simulink model "vehicle_hostmodel_2022b_Vignesh"  (R2022b)
settings: Solver=VariableStepAuto  StartTime=0  StopTime=1000  RelTol=1e-3
model workspace (MAT data in the model file):
  finalint = 0
  firstWarning = 1
  originalScenarioChecksum = '114339432DE22364D47BB28FC96DC10C'
undefined symbols (not defined in the file): Acceleration, ActorID, AngularVelocity, cameraParams, curvature, DefaultGear, DEND_B, DEND_S, DEND_T, direction, DiscIntNeverNeededParam, driving, gradbp, L, LF, LR, m, matlabshared, MAX_BRAKE, MAX_STEER, MAX_TORQUE, MCAR, MIN_BRAKE, MIN_STEER, MIN_TORQUE, n, NUMD_B, NUMD_S, NUMD_T, Pitch, Pose, Position, psi_o, R, Roll, RRdamp, SceneInfo, sigbuilder_block, STEER_RATIO, stopSign_ID, Tdead, thetaRefs, TL_ID, trackingParams, TrackWidth, Ts, ts, Vdead, Velocity, WB, X_o, xRef2s, Y_o, Yaw, yRef2, yRef2s
libraries: drivingscenarioandsensors x11, simulink x10, roadrunnerscenario x9, slrealtimeutilitieslib x7, slrealtimeiplib x7, simulink_extras x5, drivingvehiclecontroller x3, trackingutilitieslib x3, robotalgslib x2, slpidlib x2, drivinglib x2, eeGeneralControl x1
(part 1 of 5)
settings Model: Creator=akshran  LastModifiedBy=giridhar.9a
settings DataIOCC: SignalLogging=off
settings DebuggingCC: UnconnectedInputMsg=warning  UnconnectedOutputMsg=warning  UnconnectedLineMsg=warning  UnderSpecifiedDimensionMsg=warning
settings ModelReferenceCC: EnableRefExpFcnMdlSchedulingChecks=on
settings RTWCC: DLArmComputeVersion=19.05

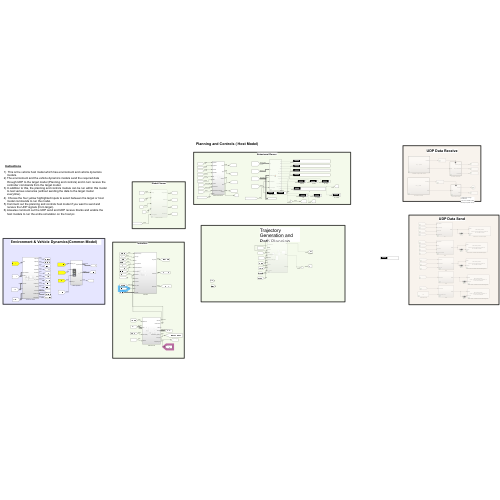
[thumbnail: Simulink's stored preview of the top-level diagram]
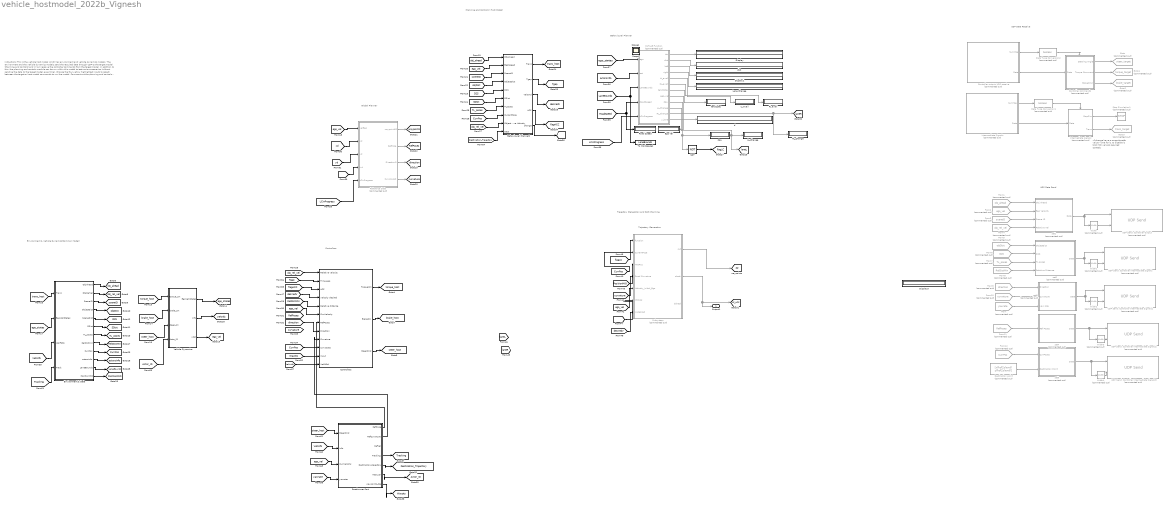
== system vehicle_hostmodel_2022b_Vignesh ==
  note: Trajectory Generation and Path Planning
  note: Global Planner
  note: xf change have a range
      | ttc safe value
      | - time for lc, to disable lc blok
      |
      | MIO vel pos required correctly
  note: Trajectory Generation
  note: Behavioural Planner
  note: Instructions
      |
      | This is the vehicle host model which has environment and vehicle dynamics models.
      | The environment and the vehicle dynamics models send the required data through UDP to the target model (Planning and controls) and in turn receive the controller commands from the target model.
      | In addition to this, the planning and controls module can be run within this model to test various scenarios (without sending the data to the target model everytime).
      | Choose the four yellow highlighted inputs to select between the target or host model commands to run the model.
      | Comment out the planning and controls host model if you want to send and receive the UDP signals (from target).
      | Likewise comment out the UDP send and UDP receive blocks and enable the host models to run the entire simulation on the host pc.
  note: Environment & Vehicle Dynamics(Common Model)
  note: UDP Data Receive
  note: UDP Data Send
  note: Planning and Controls ( Host Model)
  note: Controllers
  Behavioural Planner2 : Subsystem
  Controller commands : Subsystem  Commented=on
  Controller output- UDP receive : Subsystem  Commented=on
  Controllers : Subsystem
  Data Type Conversion1 : DataTypeConversion  Commented=on  OutDataTypeStr=boolean  SaturateOnIntegerOverflow=off  RndMeth=Floor
  Data Type Conversion2 : DataTypeConversion  Commented=on  OutDataTypeStr=boolean  SaturateOnIntegerOverflow=off  RndMeth=Floor
  Destination point : Constant  Commented=on  Value=[xRef2s(end) yRef2s(end)]
  Display : Display
  Display1 : Display
  Display3 : Display
  Ego Vel : Display
  Environment & Data : Subsystem
  From : From  Commented=on  GotoTag=yawrate  TagVisibility=global
  From1 : From  Commented=on  GotoTag=obj_ahead  TagVisibility=global
  From10 : From  Commented=on  GotoTag=curvature  TagVisibility=global
  From11 : From  Commented=on  GotoTag=RefPoses  TagVisibility=global
  From12 : From  Commented=on  GotoTag=CurrPos  TagVisibility=global
  From2 : From  Commented=on  GotoTag=ego_vel  TagVisibility=global
  From3 : From  Commented=on  GotoTag=sceneID  TagVisibility=global
  From4 : From  Commented=on  GotoTag=obj_rel_vel  TagVisibility=global
  From5 : From  Commented=on  GotoTag=objDist  TagVisibility=global
  From6 : From  Commented=on  GotoTag=D2S  TagVisibility=global
  From7 : From  Commented=on  GotoTag=TL_poses  TagVisibility=global
  From8 : From  Commented=on  GotoTag=RelDistMin  TagVisibility=global
  From9 : From  Commented=on  GotoTag=direction  TagVisibility=global
  Goto : Goto  Commented=on  GotoTag=steer_target  TagVisibility=global
  Goto1 : Goto  Commented=on  GotoTag=torque_target  TagVisibility=global
  Goto2 : Goto  Commented=on  GotoTag=brake_target  TagVisibility=global
  Goto3 : Goto  Commented=on  GotoTag=trans_target  TagVisibility=global
  Intermediate Signals : Subsystem  Commented=on
  Intermediate signals : Subsystem  Commented=on
  LL avail : Display
  LL_Change : Display
  "Lane Change " : Display
  MATLAB Function : MATLAB Function  Commented=on  TreatAsAtomicUnit=on
  NOT : Logic  Operator=NOT  IconShape=distinctive  AllPortsSameDT=off  OutDataTypeStr=boolean
  RL avail : Display
  RL_Change : Display
  Reference Data : Subsystem  Commented=on  VariantControl=Stanley
  Road Speed : Display
  Roadrunner Port : Subsystem
  Stop Simulation1 : Stop  Commented=on
  Subsystem : Subsystem  Commented=on
  To Workspace1 : ToWorkspace  VariableName=LaneBounds  SaveFormat=Timeseries  SampleTime=-1
  UDP Send: Controller Intermediate Signals : slrealtimeiplib/UDP Send  Commented=on  useHostTargetConn=on  toAddress=192.168.7.2  toPort=8002  sampleTime=0.1  enableMessage=off  ipAddress=192.168.7.2  localPort=-1
  UDP Send: Controller Intermediate Signals1 : slrealtimeiplib/UDP Send  Commented=on  useHostTargetConn=on  toAddress=192.168.7.2  toPort=8003  sampleTime=0.1  enableMessage=off  ipAddress=192.168.7.2  localPort=-1
  UDP Send: Controller Intermediate Signals2 : slrealtimeiplib/UDP Send  Commented=on  useHostTargetConn=on  toAddress=192.168.7.2  toPort=8004  sampleTime=0.1  enableMessage=off  ipAddress=192.168.7.2  localPort=-1
  UDP Send: Controller Intermediate Signals3 : slrealtimeiplib/UDP Send  Commented=on  useHostTargetConn=on  toAddress=192.168.7.2  toPort=8005  sampleTime=0.1  enableMessage=off  ipAddress=192.168.7.2  localPort=-1
  UDP Send: Controller Output : slrealtimeiplib/UDP Send  Commented=on  useHostTargetConn=on  toAddress=192.168.7.2  toPort=8001  sampleTime=0.1  enableMessage=off  ipAddress=192.168.7.2  localPort=-1
  Vehicle Dynamics : Subsystem
  Width{,1..4} (5 alike) : Width  Commented=on
  d : Display
  dist : Display
  set1 : Subsystem  Commented=on
  set2 : Subsystem  Commented=on
  set3 : Subsystem  Commented=on
  set4 : Subsystem  Commented=on
  set5 : Subsystem  Commented=on
  stay : Display
  tend2stay : Display
  Output1 : Outport
  Scope : Scope
  Scope1 : Scope
  tag scope: Actor_ID=global, CurrPos=global, D2S=global, Destination_Trajectory=global, LC_ACC=global, LaneBounds=global, PP=global, PositionMIO=global, RefPoses=global, RelDistMin=global, SDist=global, TL_poses=global, Tgap=global, Tracking=global, VehInfo=global, Waypts=global, actorsInfo=global, brake_host=global, curvature=global, desiredV=global, direction=global, ego_states=global, ego_vel=global, flagACC=global, flagLC=global, laneL=global, laneR=global, objDist=global, obj_ahead=global, obj_rel_vel=global, sceneID=global, steer_host=global, torque_host=global, trans_host=global, waypoints=global
  wires:
  Width/1 -> UDP Send: Controller Output/2
  Width1/1 -> UDP Send: Controller Intermediate Signals/2
  set1/1(Data) -> Width/1, UDP Send: Controller Output/1
  set2/1(Data) -> UDP Send: Controller Intermediate Signals/1, Width1/1
  set3/1(Data) -> UDP Send: Controller Intermediate Signals1/1, Width2/1
  Width2/1 -> UDP Send: Controller Intermediate Signals1/2
  Width3/1 -> UDP Send: Controller Intermediate Signals2/2
  set4/1(Data) -> Width3/1, UDP Send: Controller Intermediate Signals2/1
  set5/1(Data) -> Width4/1, UDP Send: Controller Intermediate Signals3/1
  Width4/1 -> UDP Send: Controller Intermediate Signals3/2
  From/1 -> set3/3(yaw rate)
  Controller output- UDP receive/2(Data) -> Controller commands/1(Data)
  Controller output- UDP receive/1(NumMsg) -> Data Type Conversion2/1
  Data Type Conversion2/1 -> Controller commands/Enable
  Data Type Conversion1/1 -> Intermediate signals/Enable
  Intermediate Signals/1(NumMsg) -> Data Type Conversion1/1
  Intermediate Signals/2(Data) -> Intermediate signals/1(Data)
  Intermediate signals/1(StopSim) -> Stop Simulation1/1
  Destination point/1 -> set5/2(Destination Point)
  Controller commands/1(Steering Angle) -> Goto/1
  Controller commands/2(Torque Command) -> Goto1/1
  Controller commands/3(BrakeCmd) -> Goto2/1
  Intermediate signals/2(Trans) -> Goto3/1
  Controllers/1(TorgueCm) -> [torque_host]
  Environment & Data/1(ObjAhead) -> [obj_ahead]
  Environment & Data/2(ObjRelVel) -> [obj_rel_vel]
  Environment & Data/3(SceneID) -> [sceneID]
  Environment & Data/4(ObjectDist) -> [objDist]
  Environment & Data/6(SDist) -> [SDist]
  Environment & Data/5(SceneDist) -> [D2S]
  Environment & Data/7(TL_poses) -> [TL_poses]
  Vehicle Dynamics/1(EgoVehStates) -> [ego_states]
  Vehicle Dynamics/3(xdot) -> [ego_vel]
  Environment & Data/8(RelDistmin) -> [RelDistMin]
  Vehicle Dynamics/2(Info) -> [VehInfo]
  From1/1 -> set1/1(Obj Ahead)
  From2/1 -> set1/2(Ego Velocity)
  From3/1 -> set1/3(Scene ID)
  From4/1 -> set1/4(Relative Vel)
  From5/1 -> set2/1(ObjectDist)
  From6/1 -> set2/2(D2S)
  From7/1 -> set2/3(TL poses)
  From8/1 -> set2/4(Relative Distance)
  From9/1 -> set3/1(Direction)
  From10/1 -> set3/2(Curvature)
  From11/1 -> set4/1(Ref Poses)
  From12/1 -> set5/1(CurrPoses)
  [torque_host] -> Vehicle Dynamics/1(torque_cm)
  [brake_host] -> Vehicle Dynamics/2(brake_cm)
  [steer_host] -> Vehicle Dynamics/3(steer_cm)
  [trans_host] -> Environment & Data/1(Trans)
  [ego_states] -> Environment & Data/2(EgoVehStates)
  [obj_rel_vel] -> Controllers/1(Relative velocity)
  [RelDistMin] -> Controllers/5(Relative distance)
  [ego_vel] -> Controllers/6(CurrVelocity)
  [direction] -> Controllers/8(Direction)
  [CurrPos] -> Controllers/10(curr poses)
  [VehInfo] -> Environment & Data/3(VehFdbk)
  Environment & Data/9(CurrPos) -> [CurrPos]
  Environment & Data/10(actorsinfo) -> [actorsInfo]
  [ego_states] -> MATLAB Function/1(ego)
  [actorsInfo] -> MATLAB Function/2(act)
  MATLAB Function/1(ttc) -> Display/1
  Environment & Data/11(LaneBounds) -> [LaneBounds]
  [LaneBounds] -> MATLAB Function/3(LaneBounds), To Workspace1/1
  MATLAB Function/3(left) -> Display1/1
  MATLAB Function/4(right) -> "Lane Change "/1
  MATLAB Function/2(dist) -> dist/1
  [RoadSpeed] -> Road Speed/1, MATLAB Function/4(RoadSpeed)
  MATLAB Function/8(ego_vel) -> Ego Vel/1
  MATLAB Function/6(RL_avail) -> RL avail/1
  MATLAB Function/5(LL_avail) -> LL avail/1
  MATLAB Function/7(tend2stay) -> tend2stay/1
  MATLAB Function/9(stay) -> NOT/1, stay/1
  MATLAB Function/10(LL_Change) -> LL_Change/1, [laneL]
  MATLAB Function/11(RL_Change) -> RL_Change/1, [laneR]
  MATLAB Function/12(y_lane) -> d/1
  Environment & Data/12(PositionMIO) -> [PositionMIO]
  NOT/1 -> [flagLC]
  [desiredV] -> Controllers/4(velocity desired)
  [ego_vel] -> Reference Data/1(velEgo)
  Reference Data/1(waypointPP) -> [waypoints]
  Reference Data/2(RefPose) -> [RefPoses]
  Reference Data/3(DirectionO) -> [direction]
  [xd] -> Reference Data/2(xd)
  [yd] -> Reference Data/3(yd)
  [Waypts] -> Controllers/11(Input)
  Reference Data/4(CurvatureO) -> [curvature]
  [LCinProgress] -> Reference Data/5(LCinProgress)
  [Tgap] -> Controllers/2(Time gap)
  [flagACC] -> Controllers/3(ACC)
  [LCinProgress] -> MATLAB Function/5(LCinProgress)
  [VehInfo] -> Controllers/12(VehFdbk)
  [sceneID] -> Behavioural Planner2/3(SceneID)
  [objDist] -> Behavioural Planner2/4(ObjectDist)
  [D2S] -> Behavioural Planner2/5(D2S)
  [CurrPos] -> Behavioural Planner2/8(CurrentPose)
  [obj_ahead] -> Behavioural Planner2/1(ObjAhead)
  [ego_vel] -> Behavioural Planner2/2(EgoSpeed)
  [SDist] -> Behavioural Planner2/6(SDist)
  [TL_poses] -> Behavioural Planner2/7(TLposes)
  [obj_rel_vel] -> Behavioural Planner2/9(Object Relative Velocity)
  Behavioural Planner2/1(Trans) -> [trans_host]
  Behavioural Planner2/2(Tgap) -> [Tgap]
  Behavioural Planner2/3(VelCmd) -> [desiredV]
  Behavioural Planner2/4(ACC) -> [flagACC]
  Behavioural Planner2/5(change) -> [change]
  [change] -> Reference Data/4(In4)
  Controllers/2(BrakeCm) -> [brake_host]
  Controllers/3(SteerCmd) -> [steer_host]
  [flagLC] -> Subsystem/1(function)
  [CurrPos] -> Subsystem/2(CurrentPose)
  [PositionMIO] -> Subsystem/3(MIOPos)
  [curvature] -> Subsystem/4(Road Curvature)
  [ego_vel] -> Subsystem/5(Velocity_Initial_Ego)
  [obj_rel_vel] -> Subsystem/6(MIOVel)
  [desiredV] -> Subsystem/7(V_desired)
  Subsystem/1(out) -> [PP]
  Subsystem/2(check) -> Output1/1, [LC_ACC]
  [VehInfo] -> Roadrunner Port/2(Info)
  [steer_host] -> Roadrunner Port/1(SteerCmd)
  Roadrunner Port/4(Tracking) -> [Tracking]
  [ego_vel] -> Roadrunner Port/3(CurrVelocity)
  [yawrate] -> Roadrunner Port/4(yawrate)
  Roadrunner Port/2(RefCurvature) -> Controllers/9(Curvature)
  Roadrunner Port/1(RefPose) -> Controllers/7(RefPoses)
  [Tracking] -> Environment & Data/4(Track)
  Roadrunner Port/5(Destination_trajectory) -> [Destination_Trajectory]
  [Destination_Trajectory] -> Behavioural Planner2/10(Dest)
  Roadrunner Port/6(Actor_ID) -> [Actor_ID]
  [Actor_ID] -> Vehicle Dynamics/4(Actor_ID)
  Roadrunner Port/7(waypoints_traj) -> [Waypts]

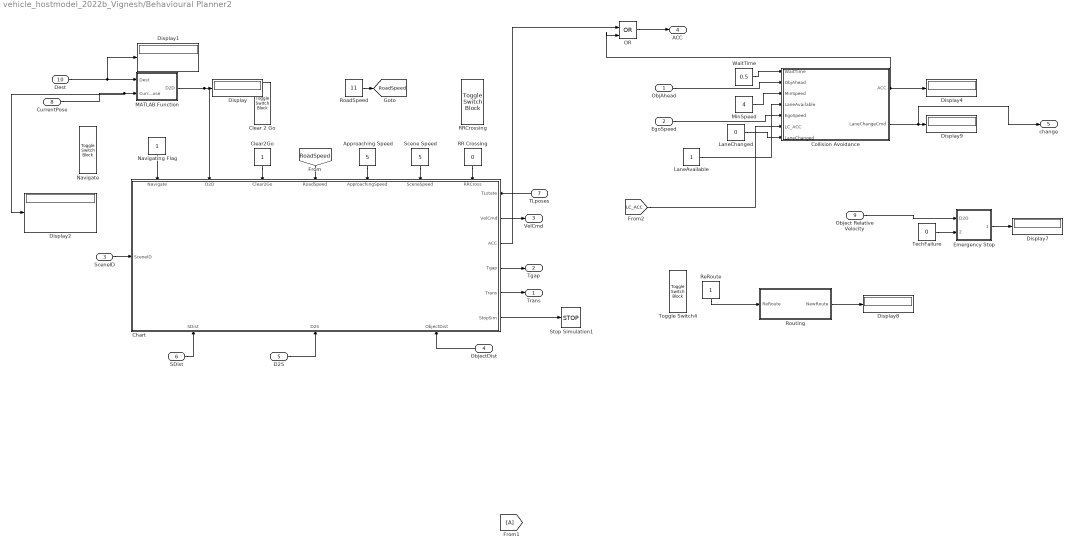
== system vehicle_hostmodel_2022b_Vignesh/Behavioural Planner2 ==
  ObjAhead : Inport
  EgoSpeed : Inport  Port=2
  SceneID : Inport  Port=3
  ObjectDist : Inport  Port=4
  D2S : Inport  Port=5
  SDist : Inport  Port=6
  TLposes : Inport  Port=7
  CurrentPose : Inport  Port=8
  Object Relative Velocity : Inport  Port=9
  Dest : Inport  Port=10
  Approaching Speed : Constant  Value=5
  Chart : Stateflow chart  TreatAsAtomicUnit=on
      settings: PortSchema="{\"entries\":[{\"content\":{\"sides\":[{\"content\":{\"connectorIds\":[\"In12\"]},\"type\":\"ConnectorPlacement.EquallySpacedRectSide\",\"uuid\":\"81aca70f-0947-49fb-b60a-be241e44193b\"},{\"content\":{\"connectorIds\":[\"In1\",\"Out1\",\"Out2\",\"Out3\",\"Out4\",\"Out5\"],\"side\":\"RIGHT\"},\"type\":\"ConnectorPlacement.EquallySpacedRectSide\",\"uuid\":\"e7b9645e-3711-4964-ac9b-0199dd335e99\"},{\"content\":{\"connectorIds\":[\"In8\",\"In9\",\"In10\",\"In11\",\"In2\",\"In4\",\"In6\"],\"side\":\"TOP\"},\"type\":\"ConnectorPlacement.EquallySpacedRectSide\",\"uuid\":\"6876f024-944b-4540-9404-d68f37763657\"},{\"content\":{\"connectorIds\":[\"In5\",\"In7\",\"In3\"],\"side\":\"BOTTOM\"},\"type\":\"ConnectorPlacement.EquallySpacedRectSide\",\"uuid\":\"44acab73-cdde-4edf-95df-27422644ccab\"}]},\"type\":\"ConnectorPlacement.EquallySpacedConnector\",\"uuid\":\"d2c31c01-e447-43db-8d2b-8b98a0ca291a\"}],\"packageUris\":[\"http://schema.mathworks.com/mf0/Connector/R2020b\"],\"version\":\"1.0\"}"
  Clear 2 Go : ToggleSwitchBlock
      settings: Values={{'Off', 'On'}, [0 1]}
  Clear2Go : Constant
  Collision Avoidance : Stateflow chart  TreatAsAtomicUnit=on
  Display{,1..2,4,7..9} (7 alike) : Display
  Emergency Stop : Stateflow chart  TreatAsAtomicUnit=on
  From1 : From
  LaneAvailable : Constant
  LaneChanged : Constant  Value=0
  MATLAB Function : MATLAB Function  TreatAsAtomicUnit=on
  MinSpeed : Constant  Value=4
  Navigate : ToggleSwitchBlock
      settings: Values={{'Off', 'On'}, [0 1]}
  Navigating Flag : Constant
  OR : Logic  Operator=OR  IconShape=distinctive  AllPortsSameDT=off  OutDataTypeStr=fixdt(1,16)
  RR Crossing : Constant  Value=0
  RRCrossing : ToggleSwitchBlock
      settings: Values={{'Off', 'On'}, [0 1]}
  ReRoute : Constant
  RoadSpeed : Constant  Value=11
  Routing : Stateflow chart  TreatAsAtomicUnit=on
  Scene Speed : Constant  Value=5
  Stop Simulation1 : Stop
  TechFailure : Constant  Value=0
  Toggle Switch4 : ToggleSwitchBlock
      settings: Values={{'Off', 'On'}, [0 1]}
  WaitTime : Constant  Value=0.5
  Trans : Outport
  Tgap : Outport  Port=2
  VelCmd : Outport  Port=3
  ACC : Outport  Port=4
  change : Outport  Port=5
  tag scope: RoadSpeed=global
  wires:
  Clear2Go/1 -> Chart/10(Clear2Go)
  Routing/1(NewRoute) -> Display8/1
  ObjectDist/1 -> Chart/3(ObjectDist)
  WaitTime/1 -> Collision Avoidance/1(WaitTime)
  Navigating Flag/1 -> Chart/8(Navigate)
  Approaching Speed/1 -> Chart/2(ApproachingSpeed)
  Scene Speed/1 -> Chart/4(SceneSpeed)
  EgoSpeed/1 -> Collision Avoidance/5(EgoSpeed)
  ReRoute/1 -> Routing/1(ReRoute)
  Collision Avoidance/2(LaneChangeCmd) -> change/1, Display9/1
  LaneAvailable/1 -> Collision Avoidance/4(LaneAvailable)
  CurrentPose/1 -> Display2/1, MATLAB Function/2(CurrentPose)
  RR Crossing/1 -> Chart/6(RRCross)
  MinSpeed/1 -> Collision Avoidance/3(MinSpeed)
  LaneChanged/1 -> Collision Avoidance/7(LaneChanged)
  [RoadSpeed] -> Chart/11(RoadSpeed)
  ObjAhead/1 -> Collision Avoidance/2(ObjAhead)
  Dest/1 -> Display1/1, MATLAB Function/1(Dest)
  SceneID/1 -> Chart/12(SceneID)
  MATLAB Function/1(D2D) -> Display/1, Chart/9(D2D)
  Chart/5(StopSim) -> Stop Simulation1/1
  Chart/4(Trans) -> Trans/1
  TLposes/1 -> Chart/1(TLstate)
  Chart/1(VelCmd) -> VelCmd/1
  SDist/1 -> Chart/5(SDist)
  D2S/1 -> Chart/7(D2S)
  Chart/3(Tgap) -> Tgap/1
  TechFailure/1 -> Emergency Stop/2(TechFailure)
  Emergency Stop/1(EStop) -> Display7/1
  Object Relative Velocity/1 -> Emergency Stop/1(D2O)
  Collision Avoidance/1(ACC) -> OR/2, Display4/1
  OR/1 -> ACC/1
  Chart/2(ACC) -> OR/1
  RoadSpeed/1 -> [RoadSpeed]
  [LC_ACC] -> Collision Avoidance/6(LC_ACC)

== system vehicle_hostmodel_2022b_Vignesh/Controller commands ==
  Data : Inport
  Enable : EnablePort
  "Byte Unpacking " : slrealtimeutilitieslib/Byte Unpacking  MaskUnpackedDataTypes={'double', 'double', 'double'}  MaskUnpackedDataSizes={[1], [1], [1]}  MaskAlignment=1
  Steering Angle : Outport
  Torque Command : Outport  Port=2
  BrakeCmd : Outport  Port=3
  wires:
  Data/1 -> "Byte Unpacking "/1
  "Byte Unpacking "/1 -> Steering Angle/1  "Steering angle"
  "Byte Unpacking "/2 -> Torque Command/1  "Longitudinal velocity"
  "Byte Unpacking "/3 -> BrakeCmd/1  "BrakeCmd"

== system vehicle_hostmodel_2022b_Vignesh/Controller output- UDP receive ==
  Compare To Constant : simulink/Logic and Bit Operations/Compare To Constant  relop===  const=24  OutDataTypeStr=boolean
  Constant : Constant
  Subtract : Sum  Inputs=+-
  UDP Receive2 : slrealtimeiplib/UDP Receive  useHostTargetConn=on  ipAddress=192.168.7.2  localPort=8016  rcvWidth=24  rcvFmAny=off  fmAddress=192.168.7.2  sampleTime=-1  enableMessage=off  maxPackets=1
  While Iterator : WhileIterator  WhileBlockType=do-while  ResetStates=reset  ShowIterationPort=on
  NumMsg : Outport
  Data : Outport  Port=2
  wires:
  Compare To Constant/1 -> While Iterator/1
  UDP Receive2/1 -> Data/1
  Constant/1 -> Subtract/2
  Subtract/1 -> NumMsg/1
  UDP Receive2/2 -> Compare To Constant/1
  While Iterator/1 -> Subtract/1

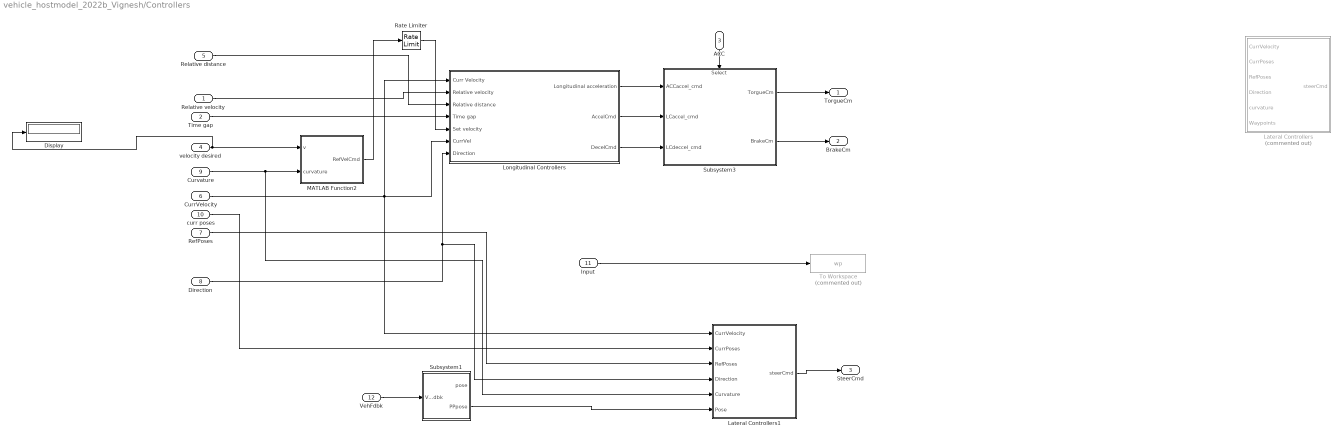
== system vehicle_hostmodel_2022b_Vignesh/Controllers ==
  Relative velocity : Inport
  Time gap : Inport  Port=2
  ACC : Inport  Port=3
  velocity desired : Inport  Port=4
  Relative distance : Inport  Port=5
  CurrVelocity : Inport  Port=6
  RefPoses : Inport  Port=7
  Direction : Inport  Port=8
  Curvature : Inport  Port=9
  curr poses : Inport  Port=10
  Input : Inport  Port=11
  VehFdbk : Inport  Port=12
  Display : Display
  Lateral Controllers : Subsystem  Commented=on
  Lateral Controllers1 : Subsystem
  Longitudinal Controllers : Subsystem
  MATLAB Function2 : MATLAB Function  TreatAsAtomicUnit=on
  Rate Limiter : RateLimiter  RisingSlewLimit=2  SampleTimeMode=inherited
  Subsystem1 : Subsystem
  Subsystem3 : Subsystem
      settings: PortSchema="{\"entries\":[{\"content\":{\"sides\":[{\"content\":{\"connectorIds\":[\"In1\",\"In2\",\"In3\"]},\"type\":\"ConnectorPlacement.EquallySpacedRectSide\",\"uuid\":\"a23b1a10-3bcb-40a0-900c-c9a3f160b173\"},{\"content\":{\"connectorIds\":[\"Out1\",\"Out2\"],\"side\":\"RIGHT\"},\"type\":\"ConnectorPlacement.EquallySpacedRectSide\",\"uuid\":\"88840b66-912f-4184-aeec-297642319416\"},{\"content\":{\"connectorIds\":[\"In4\"],\"side\":\"TOP\"},\"type\":\"ConnectorPlacement.EquallySpacedRectSide\",\"uuid\":\"37a03ca9-b065-473e-b290-3b07703c6005\"}]},\"type\":\"ConnectorPlacement.EquallySpacedConnector\",\"uuid\":\"5bfc7c71-8f7a-4cba-a168-7eeca22a2fcb\"}],\"packageUris\":[\"http://schema.mathworks.com/mf0/Connector/R2020b\"],\"version\":\"1.0\"}"
  To Workspace : ToWorkspace  Commented=on  VariableName=wp  SampleTime=-1
  TorgueCm : Outport
  BrakeCm : Outport  Port=2
  SteerCmd : Outport  Port=3
  wires:
  Longitudinal Controllers/1(Longitudinal acceleration) -> Subsystem3/1(ACCaccel_cmd)
  Curvature/1 -> MATLAB Function2/2(curvature), Lateral Controllers1/5(Curvature)
  Relative velocity/1 -> Longitudinal Controllers/2(Relative velocity)
  MATLAB Function2/1(RefVelCmd) -> Rate Limiter/1
  Direction/1 -> Longitudinal Controllers/7(Direction), Lateral Controllers1/4(Direction)
  RefPoses/1 -> Lateral Controllers1/3(RefPoses)
  velocity desired/1 -> Display/1, MATLAB Function2/1(v)
  Longitudinal Controllers/2(AccelCmd) -> Subsystem3/2(LCaccel_cmd)
  Longitudinal Controllers/3(DecelCmd) -> Subsystem3/3(LCdeccel_cmd)
  CurrVelocity/1 -> Longitudinal Controllers/1(Curr Velocity), Longitudinal Controllers/6(CurrVel), Lateral Controllers1/1(CurrVelocity)
  Time gap/1 -> Longitudinal Controllers/4(Time gap)
  Relative distance/1 -> Longitudinal Controllers/3(Relative distance)
  ACC/1 -> Subsystem3/4(Select)
  Subsystem3/1(TorgueCm) -> TorgueCm/1
  Subsystem3/2(BrakeCm) -> BrakeCm/1
  Input/1 -> To Workspace/1
  Subsystem1/2(PPpose) -> Lateral Controllers1/6(Pose)
  VehFdbk/1 -> Subsystem1/1(VehFdbk)
  Lateral Controllers1/1(steerCmd) -> SteerCmd/1
  Rate Limiter/1 -> Longitudinal Controllers/5(Set velocity)
  curr poses/1 -> Lateral Controllers1/2(CurrPoses)

== system vehicle_hostmodel_2022b_Vignesh/Environment & Data ==
  Trans : Inport
  EgoVehStates : Inport  Port=2
  VehFdbk : Inport  Port=3
  Track : Inport  Port=4
  Bus Selector4 : BusSelector  OutputSignals=Velocity,Acceleration,Position
  Sensors & Perception : Subsystem
  Subsystem1 : Subsystem
  Terminator1 : Terminator
  Terminator2 : Terminator
  Terminator3 : Terminator
  Visualisation & Data : Subsystem
  ObjAhead : Outport
  ObjRelVel : Outport  Port=2
  SceneID : Outport  Port=3
  ObjectDist : Outport  Port=4
  SceneDist : Outport  Port=5
  SDist : Outport  Port=6
  TL_poses : Outport  Port=7
  RelDistmin : Outport  Port=8
  CurrPos : Outport  Port=9
  actorsinfo : Outport  Port=10
  LaneBounds : Outport  Port=11
  PositionMIO : Outport  Port=12
  wires:
  Bus Selector4/3 -> Visualisation & Data/4(Ego Position)  "<Position>"
  Sensors & Perception/1(ObjAhead) -> ObjAhead/1
  Bus Selector4/1 -> Visualisation & Data/2(EgoVelocity)  "<Velocity>"
  Visualisation & Data/1(Actors_VehCoords) -> Sensors & Perception/1(Detections)
  Sensors & Perception/5(SceneRelVel) -> Terminator2/1
  Sensors & Perception/2(SceneAhead) -> Terminator1/1
  Sensors & Perception/6(ObjectDist) -> ObjectDist/1
  Bus Selector4/2 -> Visualisation & Data/3(Ego Acceleration)  "<Acceleration>"
  Sensors & Perception/9(ReVelmin) -> Terminator3/1
  EgoVehStates/1 -> Visualisation & Data/5(EgoInfo), Visualisation & Data/1(EgoVehStates), Sensors & Perception/2(EgoInfo), Bus Selector4/1
  Sensors & Perception/4(ObjRelVel) -> ObjRelVel/1
  Visualisation & Data/2(TL_poses) -> TL_poses/1
  Sensors & Perception/3(SceneID) -> SceneID/1
  Sensors & Perception/8(SDist) -> SDist/1
  Sensors & Perception/7(SceneDist) -> SceneDist/1
  Trans/1 -> Sensors & Perception/4(Trans)
  Sensors & Perception/10(RelDistmin) -> RelDistmin/1
  VehFdbk/1 -> Subsystem1/1(VehFdbk)
  Subsystem1/1(pose) -> CurrPos/1
  Visualisation & Data/3(actorsinfo) -> actorsinfo/1
  Visualisation & Data/4(LaneBounds) -> LaneBounds/1, Sensors & Perception/3(LaneBounds)
  Sensors & Perception/11(PositionMIO) -> PositionMIO/1
  Track/1 -> Sensors & Perception/5(Track)

== system vehicle_hostmodel_2022b_Vignesh/Intermediate Signals ==
  Compare To Constant : simulink/Logic and Bit Operations/Compare To Constant  relop===  const=16  OutDataTypeStr=boolean
  Constant : Constant
  Subtract : Sum  Inputs=+-
  UDP Receive2 : slrealtimeiplib/UDP Receive  useHostTargetConn=on  ipAddress=192.168.7.2  localPort=8017  rcvWidth=16  rcvFmAny=off  fmAddress=192.168.7.2  sampleTime=-1  enableMessage=off  maxPackets=1
  While Iterator : WhileIterator  WhileBlockType=do-while  ResetStates=reset  ShowIterationPort=on
  NumMsg : Outport
  Data : Outport  Port=2
  wires:
  While Iterator/1 -> Subtract/1
  UDP Receive2/2 -> Compare To Constant/1
  Subtract/1 -> NumMsg/1
  Constant/1 -> Subtract/2
  UDP Receive2/1 -> Data/1
  Compare To Constant/1 -> While Iterator/1

== system vehicle_hostmodel_2022b_Vignesh/Intermediate signals ==
  Data : Inport
  Enable : EnablePort
  "Byte Unpacking " : slrealtimeutilitieslib/Byte Unpacking  MaskUnpackedDataTypes={'double', 'double'}  MaskUnpackedDataSizes={[1], [1]}  MaskAlignment=1
  StopSim : Outport
  Trans : Outport  Port=2
  wires:
  "Byte Unpacking "/2 -> Trans/1  "Trans"
  "Byte Unpacking "/1 -> StopSim/1  "StopSim"
  Data/1 -> "Byte Unpacking "/1

== system vehicle_hostmodel_2022b_Vignesh/Reference Data ==
  velEgo : Inport
  xd : Inport  Port=2
  yd : Inport  Port=3
  In4 : Inport  Port=4
  LCinProgress : Inport  Port=5
  Discrete-Time Integrator : DiscreteIntegrator  SampleTime=-1  ICPrevOutput=DiscIntNeverNeededParam  ICPrevScaledInput=DiscIntNeverNeededParam
  Memory : Memory
  Memory1 : Memory
  Merge : Merge
  Merge1 : Merge
  Subsystem : Subsystem
  Subsystem1 : Subsystem
  Subsystem2 : Subsystem
  Subsystem3 : Subsystem
  Switch : Switch  Criteria=u2 ~= 0  SaturateOnIntegerOverflow=off  InputSameDT=off
  Switch Case : SwitchCase  CaseConditions={1,0}  ShowDefaultCase=off
  waypointPP : Outport
  RefPose : Outport  Port=2
  DirectionO : Outport  Port=3
  CurvatureO : Outport  Port=4
  wires:
  velEgo/1 -> Subsystem3/1(VelFdbk), Subsystem2/1(VelFdbk), Discrete-Time Integrator/1
  Subsystem2/4(WayPoints) -> Merge1/1
  Merge1/1 -> waypointPP/1
  Subsystem2/1(RefPose) -> Switch/3
  Subsystem2/2(DirectionO) -> DirectionO/1
  Merge/1 -> CurvatureO/1
  Subsystem2/3(CurvatureO) -> Merge/2
  Subsystem3/1(RefPose) -> Switch/1
  Switch Case/1 -> Subsystem3/Action
  Switch Case/2 -> Subsystem2/Action
  xd/1 -> Memory/1
  yd/1 -> Memory1/1
  Memory/1 -> Subsystem3/2(xd)
  Memory1/1 -> Subsystem3/4(yd)
  Subsystem2/5(finalint) -> Subsystem3/3(finalint)
  Subsystem/1(Out1) -> Switch/2, Switch Case/1, Subsystem1/2(enable)
  LCinProgress/1 -> Subsystem/Enable
  Discrete-Time Integrator/1 -> Subsystem1/1(Integrator)
  Subsystem1/1(Ref pose) -> RefPose/1

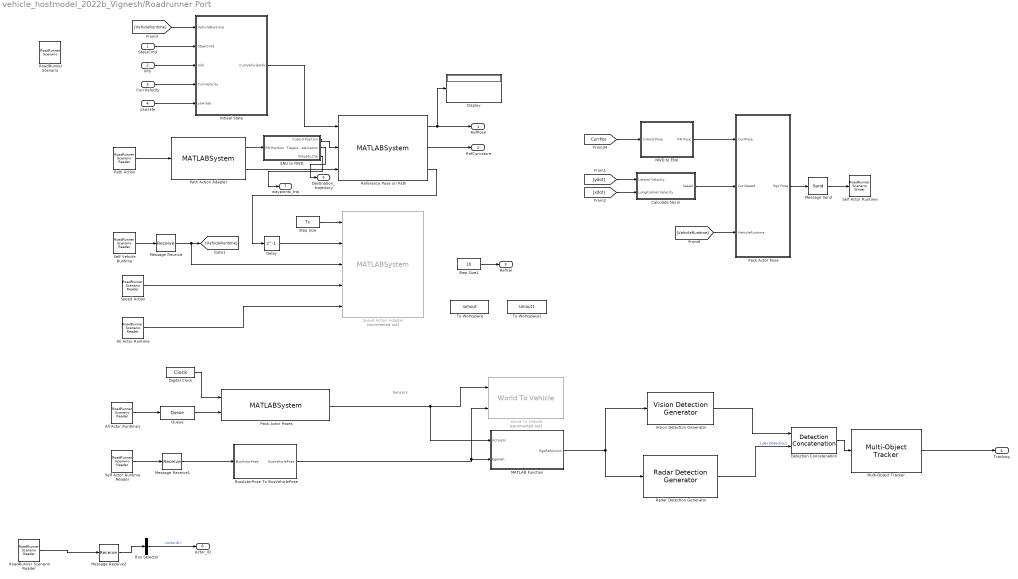
== system vehicle_hostmodel_2022b_Vignesh/Roadrunner Port ==
  note: Sensors
  SteerCmd : Inport
  Info : Inport  Port=2
  CurrVelocity : Inport  Port=3
  yawrate : Inport  Port=4
  All Actor Runtime : roadrunnerscenario/RoadRunner Scenario Reader  TopicCategory=Actor  ActorCategory=All Types  ActionType=Path Following  TopicType=Actor Pose  VehicleType=Vehicle Specifications  UserDefinedAction=Action1  Filter=None  SampleTime=Ts
  All Actor Runtime1 : roadrunnerscenario/RoadRunner Scenario Reader  TopicCategory=Actor  ActorCategory=All Types  ActionType=Path Following  TopicType=Actor Pose (Driving Scenario compatible)  VehicleType=Vehicle Specifications  UserDefinedAction=Action1  Filter=None  SampleTime=Ts
  Bus Selector : BusSelector  OutputSignals=ActorID
  BusActorPose To BusVehiclePose : Subsystem
  Calculate Norm : Subsystem
  Delay : Delay  DelayLength=1  InitialCondition=logical(0)
  Detection Concatenation : trackingutilitieslib/Detection Concatenation  NumInputs=2  BusNameSource=Auto  BusName=BusDetectionConcatenation  SimulateUsing=Code generation
  Digital Clock : DigitalClock  SampleTime=Ts
  Display : Display
  ENU to NWD : Subsystem
  Initiaal State : Subsystem
  MATLAB Function : MATLAB Function  TreatAsAtomicUnit=on
  Message Receive : Receive  InputPortMessageModes=m
  Message Receive1 : Receive  InputPortMessageModes=m  SampleTime=Ts
  Message Receive2 : Receive  InputPortMessageModes=m  SampleTime=Ts
  Message Send : Send  OutputPortMessageModes=m
  Multi-Object Tracker : drivinglib/Multi-Object Tracker  TrackerIndex=uint32( 0 )  FilterInitializationFcn=initcvekf  AssignmentThreshold=trackingParams.assigThresh  ConfirmationThreshold=[trackingParams.M,trackingParams.N]  DeletionThreshold=[trackingParams.numCoasts,trackingParams.numCoasts]  MaxNumTracks=trackingParams.numTracks  MaxNumSensors=trackingParams.numSensors  OOSMHandling=Terminate  StateParametersSimulink=struct  HasStateParametersInput=off  TimeInputSource=Auto  HasCostMatrixInput=off  HasDetectableTrackIDsInput=off  BusNameSource=Property  BusName=BusMultiObjectTracker1  TentativeTracksOutputPort=off  AllTracksOutputPort=off  SimulateUsing=Interpreted execution
  NWD to ENU : Subsystem
  Pack Actor Pose : Subsystem
  Pack Actor Poses : MATLABSystem  InputPortMessageModes=n,m  System=HelperPackDrivingScenarioPoses  EgoActorID=1  ActorProfiles=struct( 'ActorID', 1, 'ClassID', 1, 'Length', 4.7, 'Width', 1.8, 'Height', 1.4, 'OriginOffset', [ 0, 0, 0 ], 'FrontOverhang', 0, 'RearOverhang', 0, 'Wheelbase', 0, 'Color', [ 0, 0, 0 ] )  DefaultActorPoses="Simulink.Bus.createMATLABStruct( \"BusActors\" )"
      mask Type: HelperPackDrivingScenarioPoses
      mask Display:
      | disp(['HelperPack' char(10) 'DrivingScenarioPoses']);
      | port_label('input',1,'time');
      | port_label('input',2,'msgs');
      | port_label('output',1,'TargetPoses');
  Path Action : roadrunnerscenario/RoadRunner Scenario Reader  TopicCategory=Action  ActorCategory=All Types  ActionType=Path Following  TopicType=Actor Specifications  VehicleType=Vehicle Specifications  UserDefinedAction=Action1  Filter=Self  SampleTime=Ts
  Path Action Adapter : MATLABSystem  InputPortMessageModes=m  System=HelperPathActionAdapter
      mask Type: HelperPathActionAdapter
      mask Display:
      | disp(['HelperPathActionAdapter' char(10) '' char(10) '']);
      | port_label('input',1,'PathAction');
      | port_label('output',1,'Path');
      | port_label('output',2,'NumPoints');
  Queue : Queue  InputPortMessageModes=m  OutputPortMessageModes=m  OverwriteOldest=on  Capacity=maxNumActors
  Radar Detection Generator : drivingscenarioandsensors/Radar Detection Generator  SensorIndex=2  UpdateInterval=0.01  SensorLocation=[ 1.5, 0 ]  Height=0.2  Yaw=0  Pitch=0  Roll=0  BusNameSource=Auto  BusName=BusRadarDetectionGenerator  MaxNumDetectionsSource=Property  MaxNumDetections=50  DetectionCoordinates=Ego Cartesian  SimulateUsing=Interpreted execution  AzimuthResolution=4  ElevationResolution=10  RangeResolution=2.5  RangeRateResolution=0.5  AzimuthBiasFraction=0.1  ElevationBiasFraction=0.1  RangeBiasFraction=0.05  RangeRateBiasFraction=0.05  FieldOfView=[ 60, 5 ]  MaxRange=150  RangeRateLimits=[ -100, 100 ]  DetectionProbability=0.9  FalseAlarmRate=1e-6  ReferenceRange=100  ReferenceRCS=0  HasElevation=off  HasRangeRate=on  HasNoise=on  HasFalseAlarms=on  HasOcclusion=on  InitialSeedSource=Repeatable  InitialSeed=0  UsedSeed=matlabshared.tracking.internal.SimulinkUtilities.seedManager(gcb)  ActorProfilesSource=Parameters  ActorProfilesParameters=driving.internal.ActorProfilesRadarParameters  ActorProfilesExpression=struct( 'ClassID', 0, 'Length', 4.7, 'Width', 1.8, 'Height', 1.4, 'OriginOffset', [ -1.35, 0, 0 ], 'RCSPattern', [ 10, 10; 10, 10 ], 'RCSAzimuthAngles', [ -180, 180 ], 'RCSElevationAngles', [ -90, 90 ] )
  Reference Pose on Path : MATLABSystem  System=HelperReferencePoseOnPath
      mask Type: HelperReferencePoseOnPath
      mask Display:
      | disp(['HelperReferencePoseOnPath' char(10) '' char(10) '' char(10) '' char(10) '']);
      | port_label('input',1,'PrevVehicleInfo');
      | port_label('input',2,'Trajectory');
      | port_label('input',3,'NumTrajPoints');
      | port_label('output',1,'RefPointOnPath');
      | port_label('output',2,'RefCurvature');
      | port_label('output',3,'IsGoalReached');
  RoadRunner Scenario : roadrunnerscenario/RoadRunner Scenario  UserDefinedActions={}
  RoadRunner Scenario Reader : roadrunnerscenario/RoadRunner Scenario Reader  TopicCategory=Actor  ActorCategory=All Types  ActionType=Path Following  TopicType=Actor Specifications  VehicleType=Vehicle Specifications  UserDefinedAction=Action1  Filter=Self  SampleTime=0
  Self Actor Runtime : roadrunnerscenario/RoadRunner Scenario Writer  TopicCategory=Actor  ActorCategory=All Types  EventType=Action Complete  VehicleType=Vehicle Pose  TopicType=Actor Pose
  Self Actor Runtime Reader : roadrunnerscenario/RoadRunner Scenario Reader  TopicCategory=Actor  ActorCategory=All Types  ActionType=Path Following  TopicType=Actor Pose (Driving Scenario compatible)  VehicleType=Vehicle Specifications  UserDefinedAction=Action1  Filter=Self  SampleTime=Ts
  Self Vehicle Runtime : roadrunnerscenario/RoadRunner Scenario Reader  TopicCategory=Actor  ActorCategory=Vehicle  ActionType=Path Following  TopicType=Actor Specifications  VehicleType=Vehicle Pose  UserDefinedAction=Action1  Filter=Self  SampleTime=Ts
  Speed Action : roadrunnerscenario/RoadRunner Scenario Reader  TopicCategory=Action  ActorCategory=All Types  ActionType=Speed Change  TopicType=Actor Specifications  VehicleType=Vehicle Specifications  UserDefinedAction=Action1  Filter=Self  SampleTime=Ts
  Speed Action Adapter : MATLABSystem  Commented=on  InputPortMessageModes=n,n,n,m,m  System=HelperSpeedActionAdapter
      mask Type: HelperSpeedActionAdapter
      mask Display:
      | disp(['HelperSpeedActionAdapter' char(10) '' char(10) '']);
      | port_label('input',1,'timestep');
      | port_label('input',2,'stopVehicle');
      | port_label('input',3,'vehicleRuntime');
      | port_label('input',4,'msgSpeedAction');
      | port_label('input',5,'msgAllVehicleRuntime');
      | port_label('output',1,'currentSpeed');
  Step Size : Constant  Value=Ts
  Step Size1 : Constant  Value=10
  To Workspace : ToWorkspace  VariableName=simout  SaveFormat=Timeseries  SampleTime=-1
  To Workspace1 : ToWorkspace  VariableName=simout1  SaveFormat=Timeseries  SampleTime=-1
  Vision Detection Generator : drivingscenarioandsensors/Vision Detection Generator  SensorIndex=1  DetectorOutput=Objects only  UpdateInterval=Ts  LaneUpdateInterval=Ts  SensorLocation=[ 2.1, 0 ]  Height=1.1  Yaw=0  Pitch=cameraParams.pitchAngle  Roll=0  BusNameSource=Auto  BusName=BusVision  BusName2Source=Auto  BusName2=BusLaneDetections  MaxNumDetectionsSource=Property  MaxNumDetections=20  MaxNumLanesSource=Property  MaxNumLanes=30  DetectionCoordinates=Ego Cartesian  SimulateUsing=Interpreted execution  MaxRange=cameraParams.cameraRange  BoundingBoxAccuracy=5  ProcessNoiseIntensity=5  MaxSpeed=50  MaxAllowedOcclusion=0.5  MinObjectImageSize=[ 15, 15 ]  DetectionProbability=0.9  FalsePositivesPerImage=0.1  MinLaneImageSize=[ 20, 5 ]  LaneBoundaryAccuracy=3  HasNoise=on  InitialSeedSource=Repeatable  InitialSeed=0  UsedSeed=driving.internal.SimulinkUtilities.seedManager(gcb)  ActorProfilesSource=MATLAB expression  ActorProfilesParameters=driving.internal.ActorProfilesParameters  ActorProfilesExpression=actorProfiles  Intrinsics=driving.internal.cameraIntrinsics('FocalLength',cameraParams.focalLength,'PrincipalPoint',cameraParams.principalPoint,'ImageSize',cameraParams.imageSize)
  World To Vehicle : drivingscenarioandsensors/World To Vehicle  Commented=on  BusNameSource=Auto  BusName=BusWorldToVehicleActors  SimulateUsing=Interpreted execution
  RefPose : Outport
  RefCurvature : Outport  Port=2
  RefVel : Outport  Port=3
  Tracking : Outport  Port=4
  Destination_trajectory : Outport  Port=5
  Actor_ID : Outport  Port=6
  waypoints_traj : Outport  Port=7
  wires:
  Delay/1 -> Speed Action Adapter/2
  Reference Pose on Path/3 -> Delay/1
  Path Action Adapter/1 -> ENU to NWD/1(RR Position)
  Step Size/1 -> Speed Action Adapter/1
  Self Vehicle Runtime/1 -> Message Receive/1
  Message Receive/1 -> Speed Action Adapter/3, [VehicleRuntime]
  Path Action Adapter/2 -> Reference Pose on Path/3
  Path Action/1 -> Path Action Adapter/1
  ENU to NWD/1(Cuboid Position) -> Reference Pose on Path/2
  Initiaal State/1(CurrVehicleInfo) -> Reference Pose on Path/1
  [VehicleRuntime] -> Initiaal State/1(VehicleRuntime)
  SteerCmd/1 -> Initiaal State/2(SteerCmd)
  Info/1 -> Initiaal State/3(Info)
  CurrVelocity/1 -> Initiaal State/4(CurrVelocity)
  yawrate/1 -> Initiaal State/5(yawrate)
  Reference Pose on Path/1 -> RefPose/1, Display/1
  Reference Pose on Path/2 -> RefCurvature/1
  Message Send/1 -> Self Actor Runtime/1
  [CurrPos] -> NWD to ENU/1(Cuboid Pose)
  [ydot] -> Calculate Norm/1(Lateral Velocity)
  [xdot] -> Calculate Norm/2(Longitudinal Velocity)
  Calculate Norm/1(Speed) -> Pack Actor Pose/2(CurrSpeed)
  NWD to ENU/1(RR Pose) -> Pack Actor Pose/1(CurrPose)
  [VehicleRuntime] -> Pack Actor Pose/3(VehicleRuntime)
  Pack Actor Pose/1(Ego Pose) -> Message Send/1
  Pack Actor Poses/1 -> MATLAB Function/1(ActorsIn), World To Vehicle/1
  Queue/1 -> Pack Actor Poses/2
  Digital Clock/1 -> Pack Actor Poses/1
  Self Actor Runtime Reader/1 -> Message Receive1/1
  Message Receive1/1 -> BusActorPose To BusVehiclePose/1(BusActorPose)
  All Actor Runtime1/1 -> Queue/1
  Step Size1/1 -> RefVel/1
  Speed Action/1 -> Speed Action Adapter/4
  All Actor Runtime/1 -> Speed Action Adapter/5
  BusActorPose To BusVehiclePose/1(BusVehiclePose) -> MATLAB Function/2(EgoVeh), World To Vehicle/2
  Detection Concatenation/1 -> Multi-Object Tracker/1
  Radar Detection Generator/1 -> Detection Concatenation/2  "Lidar Detections"
  Vision Detection Generator/1 -> Detection Concatenation/1
  MATLAB Function/1(EgoRefActors) -> Radar Detection Generator/1, Vision Detection Generator/1
  Multi-Object Tracker/1 -> Tracking/1
  ENU to NWD/2(Trajectory Destination) -> Destination_trajectory/1
  RoadRunner Scenario Reader/1 -> Message Receive2/1
  Message Receive2/1 -> Bus Selector/1
  Bus Selector/1 -> Actor_ID/1  "<ActorID>"
  ENU to NWD/3(Waypts_traj) -> waypoints_traj/1

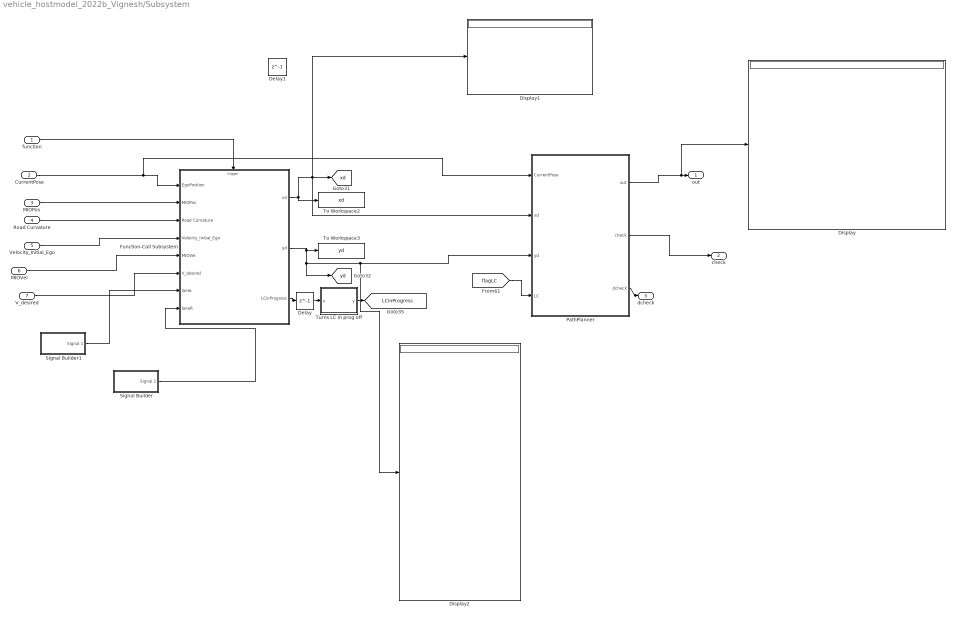
== system vehicle_hostmodel_2022b_Vignesh/Subsystem ==
  function : Inport
  CurrentPose : Inport  Port=2
  MIOPos : Inport  Port=3
  Road Curvature : Inport  Port=4
  Velocity_Initial_Ego : Inport  Port=5
  MIOVel : Inport  Port=6
  V_desired : Inport  Port=7
  Delay : Delay  DelayLength=1
  Delay1 : Delay  DelayLength=1
  Display : Display
  Display1 : Display
  Display2 : Display
  Function-Call Subsystem : Subsystem  TreatAsAtomicUnit=on
  PathPlanner : Subsystem
  Signal Builder : Subsystem  Tag=STV Subsys  LoadFcn=sigbuilder_block('load');  StartFcn=sigbuilder_block('start');  StopFcn=sigbuilder_block('stop');  ClipboardFcn=sigbuilder_block('clipboard');  mask(Sigbuilder block){tuvar=[0:10]}
      mask help: Simulink:masks:SigbuilderBlock_MD
      mask init:
      | if ~strcmp(get_param(bdroot(gcbh),'SimulationStatus'),'stopped') tuvar = sigbuilder_block('maskInit'); end
      settings: CopyFcn=sigbuilder_block('copy');  DeleteFcn=sigbuilder_block('delete');  ModelCloseFcn=sigbuilder_block('modelClose');  PreSaveFcn=sigbuilder_block('preSave');  PauseFcn=sigbuilder_block('pause');  ContinueFcn=sigbuilder_block('continue');  NameChangeFcn=sigbuilder_block('namechange');  OpenFcn=sigbuilder_block('open',[437.6 199.2 550.4 400 ]);  CloseFcn=sigbuilder_block('close');
      mask Display: plot(0, 0, 100, 100,[2, 2, 32, 32, 2], [68, 8, 8, 68, 68],[32, 2], [38, 38], [32, 19, 2],[53, 60, 44], [32, 17, 17, 2],[16, 16, 31, 31]);txt = getActiveGroup(gcbh);text(2, 100, txt,'verticalAlignment', 'top');
  Signal Builder1 : Subsystem  Tag=STV Subsys  LoadFcn=sigbuilder_block('load');  StartFcn=sigbuilder_block('start');  StopFcn=sigbuilder_block('stop');  ClipboardFcn=sigbuilder_block('clipboard');  mask(Sigbuilder block){tuvar=[0:10]}
      mask help: Simulink:masks:SigbuilderBlock_MD
      mask init:
      | if ~strcmp(get_param(bdroot(gcbh),'SimulationStatus'),'stopped') tuvar = sigbuilder_block('maskInit'); end
      settings: CopyFcn=sigbuilder_block('copy');  DeleteFcn=sigbuilder_block('delete');  ModelCloseFcn=sigbuilder_block('modelClose');  PreSaveFcn=sigbuilder_block('preSave');  PauseFcn=sigbuilder_block('pause');  ContinueFcn=sigbuilder_block('continue');  NameChangeFcn=sigbuilder_block('namechange');  OpenFcn=sigbuilder_block('open',[437.6 199.2 550.4 400 ]);  CloseFcn=sigbuilder_block('close');
      mask Display: plot(0, 0, 100, 100,[2, 2, 32, 32, 2], [68, 8, 8, 68, 68],[32, 2], [38, 38], [32, 19, 2],[53, 60, 44], [32, 17, 17, 2],[16, 16, 31, 31]);txt = getActiveGroup(gcbh);text(2, 100, txt,'verticalAlignment', 'top');
  To Workspace2 : ToWorkspace  VariableName=xd  SampleTime=-1
      settings: Save2DSignal=2-D array (concatenate along first dimension)
  To Workspace3 : ToWorkspace  VariableName=yd  SampleTime=-1
      settings: Save2DSignal=2-D array (concatenate along first dimension)
  Turns LC in prog off : MATLAB Function  TreatAsAtomicUnit=on
  out : Outport
  check : Outport  Port=2
  dcheck : Outport  Port=3
  tag scope: LCinProgress=global, xd=global, yd=global
  wires:
  MIOVel/1 -> Function-Call Subsystem/5(MIOVel)
  Road Curvature/1 -> Function-Call Subsystem/3(Road Curvature)
  PathPlanner/1(out) -> Display/1, out/1
  Signal Builder/1(Signal 1) -> Function-Call Subsystem/8(laneR)
  PathPlanner/3(dcheck) -> dcheck/1
  PathPlanner/2(check) -> check/1
  Velocity_Initial_Ego/1 -> Function-Call Subsystem/4(Velocity_Initial_Ego)
  Signal Builder1/1(Signal 1) -> Function-Call Subsystem/7(laneL)
  V_desired/1 -> Function-Call Subsystem/6(V_desired)
  MIOPos/1 -> Function-Call Subsystem/2(MIOPos)
  Function-Call Subsystem/1(xd) -> To Workspace2/1, PathPlanner/2(xd), [xd], Display1/1
  Function-Call Subsystem/2(yd) -> Display2/1, PathPlanner/3(yd), [yd], To Workspace3/1
  [flagLC] -> PathPlanner/4(LC)
  Delay/1 -> Turns LC in prog off/1(u)
  Turns LC in prog off/1(y) -> [LCinProgress]
  Function-Call Subsystem/3(LCinProgress) -> Delay/1
  CurrentPose/1 -> PathPlanner/1(CurrentPose), Function-Call Subsystem/1(EgoPosition)
  function/1 -> Function-Call Subsystem/Trigger

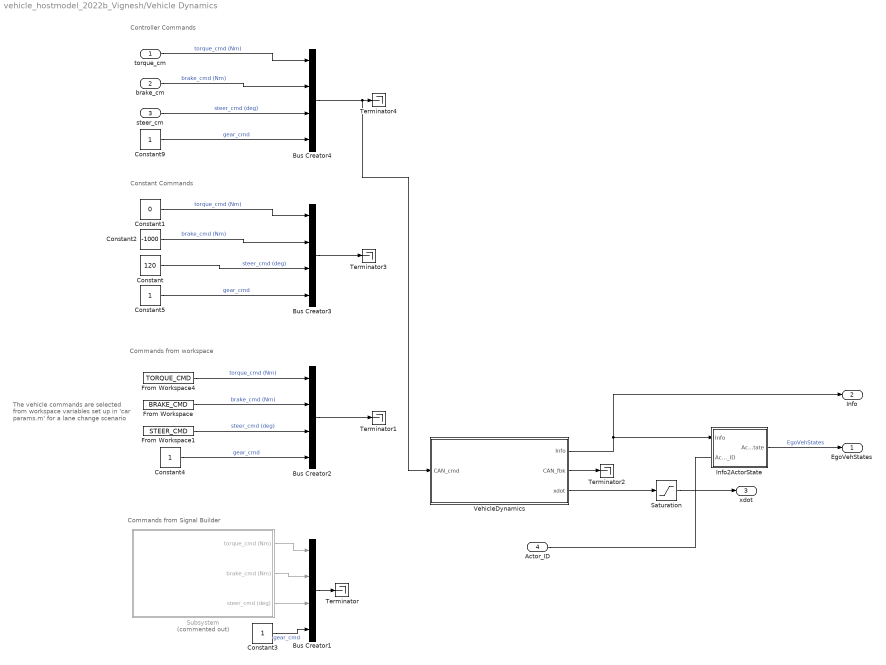
== system vehicle_hostmodel_2022b_Vignesh/Vehicle Dynamics ==
  note: Constant Commands
  note: Commands from workspace
  note: Commands from Signal Builder
  note: The vehicle commands are selected from workspace variables set up in 'car params.m' for a lane change scenario
  note: Controller Commands
  torque_cm : Inport
  brake_cm : Inport  Port=2
  steer_cm : Inport  Port=3
  Actor_ID : Inport  Port=4
  Bus Creator{1..4} (4 alike) : BusCreator  Inputs=4
  Constant : Constant  Value=120
  Constant1 : Constant  Value=0
  Constant2 : Constant  Value=-1000
  Constant{3..5,9} (4 alike) : Constant
  From Workspace : FromWorkspace  VariableName=BRAKE_CMD  SampleTime=ts
  From Workspace1 : FromWorkspace  VariableName=STEER_CMD  SampleTime=ts
  From Workspace4 : FromWorkspace  VariableName=TORQUE_CMD  SampleTime=ts
  Info2ActorState : Subsystem
  Saturation : Saturate  UpperLimit=inf  LowerLimit=0.001
  Subsystem : Subsystem  Commented=on
  Terminator{,1..4} (5 alike) : Terminator
  VehicleDynamics : Subsystem  mask{InitPosition=[X_o Y_o 0], InitSpeed=0, InitYaw=psi_o}
      mask prompts: InitPosition "Initial Position (m)"; InitSpeed "Initial Speed (m/s)"; InitYaw "Init Yaw (rad)"
  EgoVehStates : Outport
  Info : Outport  Port=2
  xdot : Outport  Port=3
  wires:
  Bus Creator2/1 -> Terminator1/1
  VehicleDynamics/2(CAN_fbk) -> Terminator2/1
  VehicleDynamics/1(Info) -> Info/1, Info2ActorState/1(Info)
  Constant/1 -> Bus Creator3/3  "steer_cmd (deg)"
  Info2ActorState/1(ActorState) -> EgoVehStates/1  "EgoVehStates"
  Constant1/1 -> Bus Creator3/1  "torque_cmd (Nm)"
  Constant2/1 -> Bus Creator3/2  "brake_cmd (Nm)"
  VehicleDynamics/3(xdot) -> Saturation/1
  Subsystem/1(torque_cmd (Nm)) -> Bus Creator1/1
  Subsystem/2(brake_cmd (Nm)) -> Bus Creator1/2
  Subsystem/3(steer_cmd (deg)) -> Bus Creator1/3
  Constant3/1 -> Bus Creator1/4  "gear_cmd"
  Constant4/1 -> Bus Creator2/4  "gear_cmd"
  From Workspace/1 -> Bus Creator2/2  "brake_cmd (Nm)"
  From Workspace1/1 -> Bus Creator2/3  "steer_cmd (deg)"
  From Workspace4/1 -> Bus Creator2/1  "torque_cmd (Nm)"
  Constant5/1 -> Bus Creator3/4  "gear_cmd"
  Bus Creator1/1 -> Terminator/1
  brake_cm/1 -> Bus Creator4/2  "brake_cmd (Nm)"
  Constant9/1 -> Bus Creator4/4  "gear_cmd"
  torque_cm/1 -> Bus Creator4/1  "torque_cmd (Nm)"
  steer_cm/1 -> Bus Creator4/3  "steer_cmd (deg)"
  Bus Creator3/1 -> Terminator3/1
  Bus Creator4/1 -> VehicleDynamics/1(CAN_cmd), Terminator4/1
  Saturation/1 -> xdot/1
  Actor_ID/1 -> ?

== system vehicle_hostmodel_2022b_Vignesh/set1 ==
  Obj Ahead : Inport
  Ego Velocity : Inport  Port=2
  Scene ID : Inport  Port=3
  Relative Vel : Inport  Port=4
  Byte Packing : slrealtimeutilitieslib/Byte Packing  MaskPackedDataType=uint8  MaskUnpackedDataTypes={'double', 'double','double','double'}  MaskAlignment=1
  Data : Outport
  wires:
  Ego Velocity/1 -> Byte Packing/2
  Byte Packing/1 -> Data/1
  Obj Ahead/1 -> Byte Packing/1
  Scene ID/1 -> Byte Packing/3
  Relative Vel/1 -> Byte Packing/4

== system vehicle_hostmodel_2022b_Vignesh/set2 ==
  ObjectDist : Inport
  D2S : Inport  Port=2
  TL poses : Inport  Port=3
  Relative Distance : Inport  Port=4
  Byte Packing1 : slrealtimeutilitieslib/Byte Packing  MaskPackedDataType=uint8  MaskUnpackedDataTypes={'double', 'double','double','double'}  MaskAlignment=1
  Data : Outport
  wires:
  Byte Packing1/1 -> Data/1
  ObjectDist/1 -> Byte Packing1/1
  D2S/1 -> Byte Packing1/2
  TL poses/1 -> Byte Packing1/4
  Relative Distance/1 -> Byte Packing1/3

== system vehicle_hostmodel_2022b_Vignesh/set3 ==
  Direction : Inport
  Curvature : Inport  Port=2
  yaw rate : Inport  Port=3
  Byte Packing1 : slrealtimeutilitieslib/Byte Packing  MaskPackedDataType=uint8  MaskUnpackedDataTypes={'double', 'double', 'double'}  MaskAlignment=1
  Data : Outport
  wires:
  Curvature/1 -> Byte Packing1/2
  Direction/1 -> Byte Packing1/1
  Byte Packing1/1 -> Data/1
  yaw rate/1 -> Byte Packing1/3

== system vehicle_hostmodel_2022b_Vignesh/set4 ==
  Ref Poses : Inport
  Byte Packing1 : slrealtimeutilitieslib/Byte Packing  MaskPackedDataType=uint8  MaskUnpackedDataTypes={'double'}  MaskAlignment=1
  Data : Outport
  wires:
  Byte Packing1/1 -> Data/1
  Ref Poses/1 -> Byte Packing1/1

== system vehicle_hostmodel_2022b_Vignesh/set5 ==
  CurrPoses : Inport
  Destination Point : Inport  Port=2
  Byte Packing1 : slrealtimeutilitieslib/Byte Packing  MaskPackedDataType=uint8  MaskUnpackedDataTypes={'double','double'}  MaskAlignment=1
  Data : Outport
  wires:
  CurrPoses/1 -> Byte Packing1/1
  Byte Packing1/1 -> Data/1
  Destination Point/1 -> Byte Packing1/2

== system vehicle_hostmodel_2022b_Vignesh/Controllers/Lateral Controllers ==
  note: include toggle logic
  CurrVelocity : Inport
  CurrPoses : Inport  Port=2
  RefPoses : Inport  Port=3
  Direction : Inport  Port=4
  curvature : Inport  Port=5
  Waypoints : Inport  Port=6
  Constant5 : Constant  Value=0
  Gain1 : Gain  Gain=180/pi
  Gain2 : Gain  Gain=1/STEER_RATIO
  Lateral Controller Stanley : drivingvehiclecontroller/Lateral Controller Stanley  ModelType=Dynamic bicycle model  PositionGainF=2.5  PositionGainR=2.5  YawRateGain=0.2  DelayGain=0.2  VehicleMass=MCAR  Lf=LF  Lr=LR  TireStiffness=5e3  Wheelbase=3  MaxSteeringAngle=80
  Pure Pursuit Controller1 : Subsystem
  Subsystem1 : Subsystem
  Switch : Switch  Criteria=u2 > Threshold  SaturateOnIntegerOverflow=off  InputSameDT=off
  Toggle Switch1 : ToggleSwitchBlock
      settings: Values={{'Off', 'On'}, [0 1]}
  Unit Delay : UnitDelay  SampleTime=-1  HasFrameUpgradeWarning=on
  steerCmd : Outport
  wires:
  Direction/1 -> Lateral Controller Stanley/4
  [yawrate] -> Gain1/1
  CurrPoses/1 -> Pure Pursuit Controller1/1(currentPose), Subsystem1/1(pose), Lateral Controller Stanley/2
  Gain1/1 -> Lateral Controller Stanley/6
  CurrVelocity/1 -> Subsystem1/2(velocity), Lateral Controller Stanley/3
  RefPoses/1 -> Lateral Controller Stanley/1
  Switch/1 -> Gain2/1
  Lateral Controller Stanley/1 -> Switch/1, Unit Delay/1
  Constant5/1 -> Switch/2
  Gain2/1 -> steerCmd/1
  Waypoints/1 -> Subsystem1/3(Input), Pure Pursuit Controller1/2(Waypoints)
  Subsystem1/1(steerCmd) -> Switch/3
  Unit Delay/1 -> Lateral Controller Stanley/7
  curvature/1 -> Lateral Controller Stanley/5

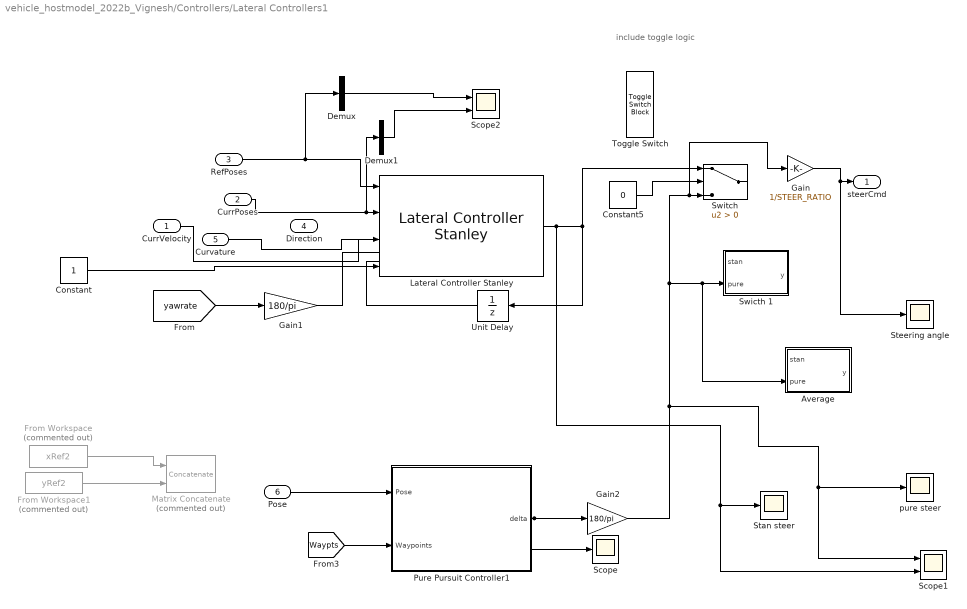
== system vehicle_hostmodel_2022b_Vignesh/Controllers/Lateral Controllers1 ==
  note: include toggle logic
  CurrVelocity : Inport
  CurrPoses : Inport  Port=2
  RefPoses : Inport  Port=3
  Direction : Inport  Port=4
  Curvature : Inport  Port=5
  Pose : Inport  Port=6
  Average : MATLAB Function  TreatAsAtomicUnit=on
  Constant : Constant
  Constant5 : Constant  Value=0
  Demux : Demux  Outputs=3
  Demux1 : Demux  Outputs=3
  From Workspace : FromWorkspace  Commented=on  VariableName=xRef2
  From Workspace1 : FromWorkspace  Commented=on  VariableName=yRef2
  Gain : Gain  Gain=1/STEER_RATIO
  Gain1 : Gain  Gain=180/pi
  Gain2 : Gain  Gain=180/pi
  Lateral Controller Stanley : drivingvehiclecontroller/Lateral Controller Stanley  ModelType=Kinematic bicycle model  PositionGainF=0.75  PositionGainR=2.5  YawRateGain=0.05  DelayGain=0.05  VehicleMass=MCAR  Lf=LF  Lr=LR  TireStiffness=5e3  Wheelbase=3  MaxSteeringAngle=30
  Matrix Concatenate : Concatenate  Commented=on  Mode=Multidimensional array  ConcatenateDimension=2
  Pure Pursuit Controller1 : Subsystem
  Scope : Scope
  Scope1 : Scope  NumInputPorts=2
  Scope2 : Scope  NumInputPorts=2
  Stan steer : Scope
  Steering angle : Scope
  Swicth 1 : MATLAB Function  TreatAsAtomicUnit=on
  Switch : Switch  Criteria=u2 > Threshold  SaturateOnIntegerOverflow=off  InputSameDT=off
  Toggle Switch : ToggleSwitchBlock
      settings: Values={{'Off', 'On'}, [0 1]}
  Unit Delay : UnitDelay  SampleTime=-1  HasFrameUpgradeWarning=on
  pure steer : Scope
  steerCmd : Outport
  wires:
  [yawrate] -> Gain1/1
  Constant5/1 -> Switch/2
  Unit Delay/1 -> ?
  CurrPoses/1 -> Demux1/1, Lateral Controller Stanley/2
  Gain1/1 -> ?
  Pure Pursuit Controller1/1(delta) -> Scope/1, Gain2/1
  Gain/1 -> Steering angle/1, steerCmd/1
  Curvature/1 -> ?
  CurrVelocity/1 -> Lateral Controller Stanley/3
  RefPoses/1 -> Demux/1, Lateral Controller Stanley/1
  Pose/1 -> Pure Pursuit Controller1/1(Pose)
  Lateral Controller Stanley/1 -> Scope1/2, Stan steer/1, Switch/1, Unit Delay/1
  Gain2/1 -> Gain/1, Switch/3, Average/2(pure), Swicth 1/2(pure), Scope1/1, pure steer/1
  From Workspace/1 -> Matrix Concatenate/1
  From Workspace1/1 -> Matrix Concatenate/2
  Constant/1 -> Lateral Controller Stanley/4
  Demux1/2 -> Scope2/2
  Demux/2 -> Scope2/1
  [Waypts] -> Pure Pursuit Controller1/2(Waypoints)
